simulink library "powerlib_extras"  (Simulink 6.0)
settings: Solver=ode45  SolverMode=SingleTasking  StartTime=0.0  StopTime=10.0  RelTol=1e-3
values from neighbouring files (symbols this model uses):
  Ts = get(handles.edit1,'string')    [powergui.m]
undefined symbols (not defined in the file or in its folder): Ac, Bc, Cc, Dc, Delay_discrete, dend, DiscIntNeverNeededParam, extra_sc, j, numd, test_alpha
libraries: powerlib2 x112, powerlib_extras x70, simulink_extras x25, simulink x12, powerlib_models x8
(part 6 of 9)

== system powerlib_extras/Measurements/dq0-based Active & Reactive Power ==
  note: 2) Q = 3/2(Vq*Id - Vd*Iq)
  note: 1) P = 3/2(Vd*Id + Vq*Iq + 2*V0*I0)
  note: This block computes the 3-phase instantaneous active and reactive power using the following equations:
  note: Note: Equation 2 is valid only for a balanced and harmonic-free system.
  note: dq0-based active and reactive power computation
  note: Gilbert Sybille, Pierre Giroux
      | Power System Simulation Laboratory
      | IREQ, Hydro-Quebc
  Vdq0 : Inport  Port=1  PortDimensions=3  LatchInput=off
  Idq0 : Inport  Port=2  PortDimensions=3  LatchInput=off
  Demux1 : Demux  Outputs=2
  Demux2 : Demux  Outputs=2
  Mux : Mux  Inputs=2
  Product{1..5} (5 alike) : Product  SaturateOnIntegerOverflow=on  InputSameDT=on
  Selector : Selector  Elements=[1 2]  InputPortWidth=3
  Selector1 : Selector  Elements=[1 2]  InputPortWidth=3
  Selector2 : Selector  Elements=3  InputPortWidth=3
  Selector3 : Selector  Elements=3  InputPortWidth=3
  Sum : Sum  Inputs=+++  SaturateOnIntegerOverflow=on  InputSameDT=on
  Sum1 : Sum  Inputs=+-  SaturateOnIntegerOverflow=on  InputSameDT=on
  pu->V1 : Gain  Gain=2  SaturateOnIntegerOverflow=on
  pu->V4 : Gain  Gain=3/2  SaturateOnIntegerOverflow=on
  PQ : Outport
  wires:
  Vdq0/1 -> Selector2/1, Selector/1
  Idq0/1 -> Selector3/1, Selector1/1
  Demux2/2 -> Product3/2, Product5/2
  Demux1/1 -> Product2/1, Product5/1
  Demux2/1 -> Product2/2, Product4/2
  Demux1/2 -> Product3/1, Product4/1
  Sum1/1 -> Mux/2
  Sum/1 -> Mux/1
  Product5/1 -> Sum1/2
  Product4/1 -> Sum1/1
  Product3/1 -> Sum/2
  Product2/1 -> Sum/1
  Selector/1 -> Demux1/1
  Selector1/1 -> Demux2/1
  Selector2/1 -> Product1/1
  Selector3/1 -> Product1/2
  Product1/1 -> pu->V1/1
  pu->V1/1 -> Sum/3
  Mux/1 -> pu->V4/1
  pu->V4/1 -> PQ/1

== system powerlib_extras/Measurements/dq0_to_abc Transformation ==
  note: Va= Vd*sinwt + Vq*cos(wt) + Vo
  note: Vb= Vd*sin(wt-2pi/3) + Vq*cos(wt-2pi/3) + Vo
  note: Vc= Vd*sin(wt+2pi/3) + Vq*cos(wt+2pi/3) + Vo
  dq0 : Inport  Port=1  PortDimensions=3  LatchInput=off
  sin_cos : Inport  Port=2  PortDimensions=2  LatchInput=off
  Demux : Demux  Outputs=2
  Fcn2 : Fcn  Expr="u[1]*u[4] +  u[2]*u[5] + u[3]"
  Fcn4 : Fcn  Expr="u[1]*u[6] +  u[2]*u[7]+ u[3]"
  Fcn5 : Fcn  Expr="u[1]*u[8]+  u[2]*u[9]+ u[3]"
  K1 : Constant  Value=0.5
  K2 : Constant  Value=sqrt(3)/2
  Mux : Mux  Inputs=2
  Mux1 : Mux  Inputs=3
  Mux2 : Mux  Inputs=6
  Product{,1..3} (4 alike) : Product  SaturateOnIntegerOverflow=on  InputSameDT=on
  Sum : Sum  Inputs=--  SaturateOnIntegerOverflow=on  InputSameDT=on
  Sum1 : Sum  Inputs=-+  SaturateOnIntegerOverflow=on  InputSameDT=on
  Sum2 : Sum  Inputs=--  SaturateOnIntegerOverflow=on  InputSameDT=on
  Sum3 : Sum  Inputs=--  SaturateOnIntegerOverflow=on  InputSameDT=on
  abc : Outport  InitialOutput=0
  wires:
  Fcn5/1 -> Mux1/3  "Vc"
  Fcn2/1 -> Mux1/1  "Va"
  Mux1/1 -> abc/1
  Mux/1 -> Fcn4/1, Fcn2/1, Fcn5/1
  Sum1/1 -> Sum3/1, Mux2/4  "cos(wt-2pi/3)"
  Sum/1 -> Sum2/1, Mux2/3  "sin(wt-2pi/3)"
  K2/1 -> Product2/2, Product1/2
  K1/1 -> Product3/2, Product/2
  Sum2/1 -> Mux2/5  "sin(wt+2pi/3)"
  Sum3/1 -> Mux2/6  "cos(wt+2pi/3)"
  Product2/1 -> Sum1/2
  Product3/1 -> Sum1/1
  Product1/1 -> Sum/2
  Product/1 -> Sum/1
  Demux/1 -> Mux2/1, Sum2/2, Product2/1, Product/1  "sin(wt)"
  Demux/2 -> Mux2/2, Product1/1, Product3/1, Sum3/2  "cos(wt)"
  sin_cos/1 -> Demux/1
  Mux2/1 -> Mux/2
  dq0/1 -> Mux/1  "Vabc"
  Fcn4/1 -> Mux1/2  "Vb"

== system powerlib_extras/Phasor Library/3-Phase Active & Reactive Power (Phasor Type) ==
  Vabc : Inport  Port=1  PortDimensions=3  LatchInput=off
  Iabc : Inport  Port=2  PortDimensions=3  LatchInput=off
  Complex to Real-Imag : ComplexToRealImag
  K : Gain  Gain=1/2  SaturateOnIntegerOverflow=on
  Math Function : Math  Operator=conj  SaturateOnIntegerOverflow=on
  Mux : Mux  Inputs=2
  Product2 : Product  SaturateOnIntegerOverflow=on  InputSameDT=on
  Sum3 : Sum  Inputs=1  SaturateOnIntegerOverflow=on  InputSameDT=on
  PQ : Outport
  wires:
  Iabc/1 -> Math Function/1
  Vabc/1 -> Product2/1
  Math Function/1 -> Product2/2
  Product2/1 -> Sum3/1
  Sum3/1 -> K/1
  K/1 -> Complex to Real-Imag/1
  Complex to Real-Imag/1 -> Mux/1
  Complex to Real-Imag/2 -> Mux/2
  Mux/1 -> PQ/1

== system powerlib_extras/Phasor Library/Active & Reactive Power (Phasor Type) ==
  V : Inport  Port=1  LatchInput=off
  I : Inport  Port=2  LatchInput=off
  Complex to Real-Imag : ComplexToRealImag
  K : Gain  Gain=1/2  SaturateOnIntegerOverflow=on
  Math Function : Math  Operator=conj  SaturateOnIntegerOverflow=on
  Mux : Mux  Inputs=2
  Product2 : Product  SaturateOnIntegerOverflow=on  InputSameDT=on
  PQ : Outport
  wires:
  I/1 -> Math Function/1
  K/1 -> Complex to Real-Imag/1
  Product2/1 -> K/1
  Math Function/1 -> Product2/2
  V/1 -> Product2/1
  Complex to Real-Imag/1 -> Mux/1
  Complex to Real-Imag/2 -> Mux/2
  Mux/1 -> PQ/1

== system powerlib_extras/Phasor Library/Mean Value (Phasor Type) ==
  note: Mean value (phasor type)
  In : Inport  Port=1  LatchInput=off
  Complex to Real-Imag : ComplexToRealImag
  Demux : Demux  Outputs=2
  Gain : Gain  Gain=1/Period  SaturateOnIntegerOverflow=on
  Mux : Mux  Inputs=2
  Real-Imag to Complex : RealImagToComplex
  Sum : Sum  Inputs=+-  SaturateOnIntegerOverflow=on  InputSameDT=on
  Transport Delay : TransportDelay  DelayTime=Period
  integrator : Integrator
  Mean : Outport
  wires:
  integrator/1 -> Transport Delay/1, Sum/1
  In/1 -> Complex to Real-Imag/1
  Complex to Real-Imag/1 -> Mux/1
  Complex to Real-Imag/2 -> Mux/2
  Gain/1 -> Demux/1
  Demux/1 -> Real-Imag to Complex/1
  Demux/2 -> Real-Imag to Complex/2
  Real-Imag to Complex/1 -> Mean/1
  Mux/1 -> integrator/1
  Transport Delay/1 -> Sum/2
  Sum/1 -> Gain/1

== system powerlib_extras/Phasor Library/Sequence Analyzer (Phasor Type) ==
  note: Negative sequence :V2 = 1/3 * (Va + a^2*Vb + a *Vc )
  note: Positive sequence :V1 = 1/3 * (Va + a*Vb + a^2 *Vc )
  note: where a =exp(j *2pi/3) = 1 < + 120 deg.
  note: Zero sequence :V0 = 1/3 * (Va + Vb + Vc )
  abc : Inport  Port=1  PortDimensions=3  LatchInput=off
  Complex to Magnitude-Angle : ComplexToMagnitudeAngle
  Constant : Constant  Value=PosOn
  Constant1 : Constant  Value=NegOn
  Constant2 : Constant  Value=ZeroOn
  Mux2 : Mux  Inputs=3
  Neg. Seq. Computation : Subsystem  TreatAsAtomicUnit=on
  Pos. Seq. Computation : Subsystem  TreatAsAtomicUnit=on
  Selector : Selector  Elements=SelectElement  InputPortWidth=3
  Selector1 : Selector  Elements=SelectElement  InputPortWidth=3
  Zero Seq. Computation : Subsystem  TreatAsAtomicUnit=on
  rad->deg1 : Gain  Gain=180/pi  SaturateOnIntegerOverflow=on
  Mag : Outport
  Pha : Outport  Port=2
  wires:
  Constant1/1 -> Neg. Seq. Computation/Enable
  Selector1/1 -> rad->deg1/1
  Constant2/1 -> Zero Seq. Computation/Enable
  Constant/1 -> Pos. Seq. Computation/Enable
  Mux2/1 -> Complex to Magnitude-Angle/1
  Zero Seq. Computation/1(Out) -> Mux2/3
  Neg. Seq. Computation/1(Out) -> Mux2/2
  Pos. Seq. Computation/1(Out) -> Mux2/1
  abc/1 -> Zero Seq. Computation/1(In), Neg. Seq. Computation/1(In), Pos. Seq. Computation/1(In)  "Vabc"
  rad->deg1/1 -> Pha/1
  Selector/1 -> Mag/1
  Complex to Magnitude-Angle/1 -> Selector/1
  Complex to Magnitude-Angle/2 -> Selector1/1

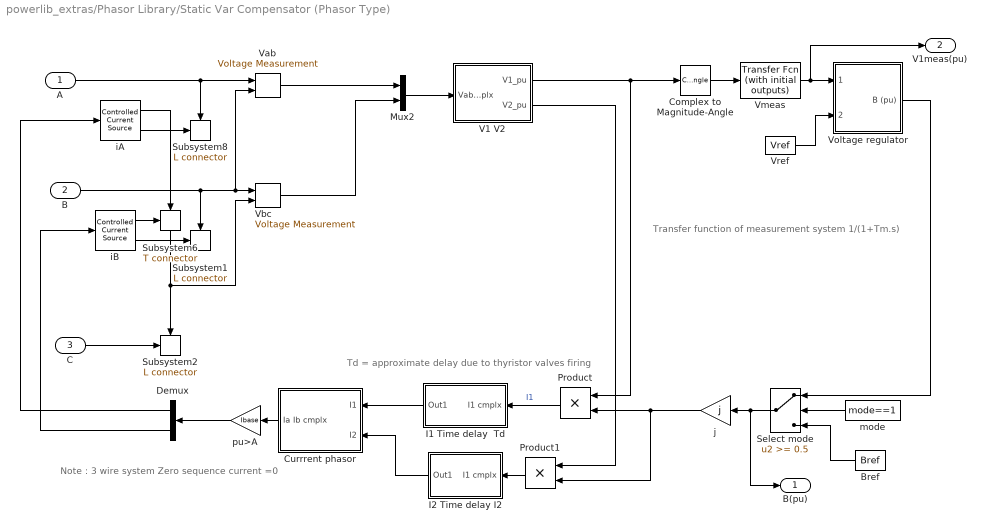
== system powerlib_extras/Phasor Library/Static Var Compensator (Phasor Type) ==
  note: Transfer function of measurement system
      | 1/(1+Tm.s)
  note: Td = approximate delay
      | due to thyristor valves firing
  note: Note : 3 wire system
      | Zero sequence current =0
  A : Inport  Port=1  LatchInput=off
  B : Inport  Port=2  LatchInput=off
  C : Inport  Port=3  LatchInput=off
  Bref : Constant  Orientation=left  Value=Bref
  Complex to Magnitude-Angle : ComplexToMagnitudeAngle  Output=Magnitude
  Currrent phasor : Subsystem  Orientation=left
  Demux : Demux  Orientation=left  Outputs=2
  I1 Time delay  Td : Subsystem  Orientation=left
  I2 Time delay I2 : Subsystem  Orientation=left
  Mux2 : Mux  Inputs=2
  Product : Product  Orientation=left  SaturateOnIntegerOverflow=on  InputSameDT=on
  Product1 : Product  Orientation=left  SaturateOnIntegerOverflow=on  InputSameDT=on
  Select mode : Switch  Orientation=left  Threshold=0.5  InputSameDT=on
  Subsystem1 : powerlib2/Connectors/L connector  Tag=PoWeRsYsTeMbLoCk
  Subsystem2 : powerlib2/Connectors/L connector  Tag=PoWeRsYsTeMbLoCk
  Subsystem6 : powerlib2/Connectors/T connector  Tag=PoWeRsYsTeMbLoCk  Orientation=down  PSBOutputType=1
  Subsystem8 : powerlib2/Connectors/L connector  Tag=PoWeRsYsTeMbLoCk
  V1 V2 : Subsystem
  Vab : powerlib2/Measurements/Voltage Measurement  Tag=PoWeRsYsTeMmEaSuReMeNt  PhasorSimulation=on  OutputType=Complex  PSBOutputType=0  PSBequivalent=0
  Vbc : powerlib2/Measurements/Voltage Measurement  Tag=PoWeRsYsTeMmEaSuReMeNt  PhasorSimulation=on  OutputType=Complex  PSBOutputType=0  PSBequivalent=0
  Vmeas : simulink_extras/Additional Linear/Transfer Fcn (with initial outputs)  N=[1]  D="[Tm  1]"  Y0=Vref  U0=Vref
  Voltage regulator : Subsystem
  Vref : Constant  Value=Vref
  iA : powerlib2/Electrical Sources/Controlled Current Source  Tag=PoWeRsYsTeMbLoCk  Description=source block  initsrc=on  srctyp=AC  ia=0  iph=0  freq=60  mesure=None  PSBOutputType=11
  iB : powerlib2/Electrical Sources/Controlled Current Source  Tag=PoWeRsYsTeMbLoCk  Description=source block  initsrc=on  srctyp=AC  ia=0  iph=0  freq=60  mesure=None  PSBOutputType=11
  j : Gain  Orientation=left  Gain=j  SaturateOnIntegerOverflow=on
  mode : Constant  Orientation=left  Value=mode==1
  pu>A : Gain  Orientation=left  Gain=Ibase  SaturateOnIntegerOverflow=on
  B(pu) : Outport
  V1meas(pu) : Outport  Port=2
  wires:
  mode/1 -> Select mode/2
  Voltage regulator/1(B (pu)) -> Select mode/1
  Bref/1 -> Select mode/3
  Select mode/1 -> B(pu)/1, j/1
  iA/2 -> Subsystem8/1
  A/1 -> Subsystem8/Enable, Vab/1
  iB/2 -> Subsystem1/1
  B/1 -> Subsystem1/Enable, Vab/2, Vbc/1
  iA/1 -> Subsystem6/1
  iB/1 -> Subsystem6/Enable
  Subsystem6/1 -> Subsystem2/Enable, Vbc/2
  C/1 -> Subsystem2/1
  Mux2/1 -> V1 V2/1(Vab Vbc cmplx)
  V1 V2/1(V1_pu) -> Complex to Magnitude-Angle/1, Product/1
  Vref/1 -> Voltage regulator/2(Vref (pu))
  Vmeas/1 -> Voltage regulator/1(V1meas (pu)), V1meas(pu)/1
  Currrent phasor/1(Ia Ib cmplx) -> pu>A/1
  I2 Time delay I2/1(Out1) -> Currrent phasor/2(I2)
  Complex to Magnitude-Angle/1 -> Vmeas/1
  Demux/1 -> iA/1
  Demux/2 -> iB/1
  Vab/1 -> Mux2/1
  Vbc/1 -> Mux2/2
  I1 Time delay  Td/1(Out1) -> Currrent phasor/1(I1)
  pu>A/1 -> Demux/1
  Product/1 -> I1 Time delay  Td/1(I1 cmplx)  "I1"
  j/1 -> Product/2, Product1/2
  V1 V2/2(V2_pu) -> Product1/1
  Product1/1 -> I2 Time delay I2/1(I1 cmplx)

== system powerlib_extras/Three-Phase Library/6 - pulse  diode  bridge ==
  A : Inport  Port=1  LatchInput=off
  B : Inport  Port=2  LatchInput=off
  C : Inport  Port=3  LatchInput=off
  Bus Bar 5 : powerlib2/Connectors/Bus Bar (thin vert)  Tag=PoWeRsYsTeMbLoCk  input=0  output=2  PSBOutputType=111111111111111111111111111111111111111111111111111111111111111111111111111111111111
  D{1..6} (6 alike) : powerlib2/Power Electronics/Diode  Tag=PoWeRsYsTeMbLoCk  Orientation=up  Ron=Ron  Lon=Lon  Vf=Vf  IC=0  Rs=Rs  Cs=Cs  PSBOutputType=10
  Subsystem11 : powerlib2/Connectors/T connector  Tag=PoWeRsYsTeMbLoCk  PSBOutputType=1
  Subsystem12 : powerlib2/Connectors/T connector  Tag=PoWeRsYsTeMbLoCk  PSBOutputType=1
  Subsystem6 : powerlib2/Connectors/T connector  Tag=PoWeRsYsTeMbLoCk  Orientation=up  PSBOutputType=1
  Subsystem7 : powerlib2/Connectors/T connector  Tag=PoWeRsYsTeMbLoCk  Orientation=up  PSBOutputType=1
  Subsystem8 : powerlib2/Connectors/T connector  Tag=PoWeRsYsTeMbLoCk  Orientation=up  PSBOutputType=1
  Terminator{,1..5} (6 alike) : Terminator
      settings: Orientation=up
  "K " : Outport  InitialOutput=0
  "A " : Outport  Port=2  InitialOutput=0
  wires:
  Bus Bar 5/2 -> "A "/1, D2/1, D6/1
  Bus Bar 5/1 -> D4/1
  D4/2 -> Terminator3/1
  D6/2 -> Terminator4/1
  D2/2 -> Terminator5/1
  D5/2 -> Terminator2/1
  D3/2 -> Terminator1/1
  D1/2 -> Terminator/1
  Subsystem12/1 -> "K "/1
  D5/1 -> Subsystem12/Enable
  Subsystem11/1 -> Subsystem12/1
  D3/1 -> Subsystem11/Enable
  D1/1 -> Subsystem11/1
  D6/1 -> Subsystem7/1
  D4/1 -> Subsystem6/1
  C/1 -> Subsystem8/Enable
  Subsystem6/1 -> D1/1
  Subsystem7/1 -> D3/1
  D2/1 -> Subsystem8/1
  Subsystem8/1 -> D5/1
  A/1 -> Subsystem6/Enable
  B/1 -> Subsystem7/Enable

== system powerlib_extras/Three-Phase Library/6 - pulse  thyristor bridge ==
  A : Inport  Port=1  LatchInput=off
  B : Inport  Port=2  LatchInput=off
  C : Inport  Port=3  LatchInput=off
  pulses : Inport  Port=4  LatchInput=off
  Bus Bar 5 : powerlib2/Connectors/Bus Bar (thin vert)  Tag=PoWeRsYsTeMbLoCk  input=0  output=2  PSBOutputType=111111111111111111111111111111111111111111111111111111111111111111111111111111111111
  Demux1 : Demux  Outputs=3
  Demux2 : Demux  Outputs=3
  Selector : Selector  Elements=[ 4 6 2]  InputPortWidth=6
  Selector1 : Selector  Elements=[ 1 3 5]  InputPortWidth=6
  Subsystem14 : powerlib2/Connectors/T connector  Tag=PoWeRsYsTeMbLoCk  PSBOutputType=1
  Subsystem15 : powerlib2/Connectors/T connector  Tag=PoWeRsYsTeMbLoCk  PSBOutputType=1
  Subsystem6 : powerlib2/Connectors/T connector  Tag=PoWeRsYsTeMbLoCk  Orientation=up  PSBOutputType=1
  Subsystem7 : powerlib2/Connectors/T connector  Tag=PoWeRsYsTeMbLoCk  Orientation=up  PSBOutputType=1
  Subsystem8 : powerlib2/Connectors/T connector  Tag=PoWeRsYsTeMbLoCk  Orientation=up  PSBOutputType=1
  Terminator{,1..5} (6 alike) : Terminator
      settings: Orientation=up
  th{1..6} (6 alike) : powerlib2/Power Electronics/Thyristor  Tag=PoWeRsYsTeMbLoCk  Orientation=up  Ron=Ron  Lon=Lon  Vf=0  IC=0  Rs=Rs  Cs=Cs  PSBOutputType=10
  "K " : Outport  InitialOutput=0
  "A " : Outport  Port=2  InitialOutput=0
  wires:
  Bus Bar 5/2 -> "A "/1, th2/1, th6/1
  Bus Bar 5/1 -> th4/1
  Subsystem6/1 -> th1/1
  th4/1 -> Subsystem6/1
  A/1 -> Subsystem6/Enable
  th4/2 -> Terminator3/1
  th6/2 -> Terminator4/1
  th2/2 -> Terminator5/1
  th5/2 -> Terminator2/1
  th3/2 -> Terminator1/1
  th1/2 -> Terminator/1
  Subsystem15/1 -> "K "/1
  th5/1 -> Subsystem15/Enable
  Subsystem14/1 -> Subsystem15/1
  th3/1 -> Subsystem14/Enable
  th1/1 -> Subsystem14/1
  th6/1 -> Subsystem7/1
  pulses/1 -> Selector/1, Selector1/1
  B/1 -> Subsystem7/Enable
  th2/1 -> Subsystem8/1
  Subsystem7/1 -> th3/1
  Demux1/3 -> th5/2
  Demux1/2 -> th3/2
  Demux1/1 -> th1/2
  Selector1/1 -> Demux1/1
  Demux2/3 -> th2/2
  Demux2/2 -> th6/2
  Demux2/1 -> th4/2
  Selector/1 -> Demux2/1
  C/1 -> Subsystem8/Enable
  Subsystem8/1 -> th5/1

== system powerlib_extras/Three-Phase Library/DYg linear transformer ==
  A1 : Inport  Port=1  LatchInput=off
  B1 : Inport  Port=2  LatchInput=off
  C1 : Inport  Port=3  LatchInput=off
  Ground : powerlib2/Connectors/Ground (input)  Tag=PoWeRsYsTeMbLoCk  Orientation=down
  Ground1 : powerlib2/Connectors/Ground (input)  Tag=PoWeRsYsTeMbLoCk  Orientation=down
  Ground2 : powerlib2/Connectors/Ground (input)  Tag=PoWeRsYsTeMbLoCk  Orientation=down
  T1 : powerlib2/Elements/Linear Transformer  Tag=PoWeRsYsTeMbLoCk  a=[pnom fnom]  b=[ u1 r1 x1]  c=[u2 r2 x2]  w3check=off  d=[u2 r2 x2]  e=rxm  mesure=None  PSBOutputType=1111
  T2 : powerlib2/Elements/Linear Transformer  Tag=PoWeRsYsTeMbLoCk  a=[pnom fnom]  b=[ u1 r1 x1]  c=[u2 r2 x2]  w3check=off  d=[u2 r2 x2]  e=rxm  mesure=None  PSBOutputType=1111
  T3 : powerlib2/Elements/Linear Transformer  Tag=PoWeRsYsTeMbLoCk  a=[pnom fnom]  b=[ u1 r1 x1]  c=[u2 r2 x2]  w3check=off  d=[u2 r2 x2]  e=rxm  mesure=None  PSBOutputType=1111
  A2 : Outport  InitialOutput=0
  B2 : Outport  Port=2  InitialOutput=0
  C2 : Outport  Port=3  InitialOutput=0
  wires:
  T1/2 -> Ground/1
  T3/2 -> Ground2/1
  T2/2 -> Ground1/1
  T3/1 -> C2/1
  T2/1 -> B2/1
  T1/1 -> A2/1
  B1/1 -> T1/2, T2/1
  A1/1 -> T3/2, T1/1
  C1/1 -> T2/2, T3/1

== system powerlib_extras/Three-Phase Library/Inductive source with neutral ==
  N : Inport  Port=1  LatchInput=off
  Branch A : powerlib2/Elements/Series RLC Branch  Tag=PoWeRsYsTeMbLoCk  a=R  b=L  c=inf  mesure=None  PSBOutputType=1
  Branch B : powerlib2/Elements/Series RLC Branch  Tag=PoWeRsYsTeMbLoCk  a=R  b=L  c=inf  mesure=None  PSBOutputType=1
  Branch C : powerlib2/Elements/Series RLC Branch  Tag=PoWeRsYsTeMbLoCk  a=R  b=L  c=inf  mesure=None  PSBOutputType=1
  Va : powerlib2/Electrical Sources/AC Voltage Source  Tag=PoWeRsYsTeMbLoCk  A=V  P=Phi  F=F  stime=0  mesure=None  PSBOutputType=1
  Vb : powerlib2/Electrical Sources/AC Voltage Source  Tag=PoWeRsYsTeMbLoCk  A=V  P=Phi-120  F=F  stime=0  mesure=None  PSBOutputType=1
  Vc : powerlib2/Electrical Sources/AC Voltage Source  Tag=PoWeRsYsTeMbLoCk  A=V  P=Phi+120  F=F  stime=0  mesure=None  PSBOutputType=1
  A : Outport
  B : Outport  Port=2
  C : Outport  Port=3
  wires:
  Branch A/1 -> A/1
  Branch B/1 -> B/1
  Branch C/1 -> C/1
  N/1 -> Vb/1, Va/1, Vc/1
  Va/1 -> Branch A/1
  Vb/1 -> Branch B/1
  Vc/1 -> Branch C/1

== system powerlib_extras/Three-Phase Library/YgD  linear transformer  ==
  A1 : Inport  Port=1  LatchInput=off
  B1 : Inport  Port=2  LatchInput=off
  C1 : Inport  Port=3  LatchInput=off
  Subsystem10 : powerlib2/Connectors/T connector  Tag=PoWeRsYsTeMbLoCk  PSBOutputType=1
  Subsystem11 : powerlib2/Connectors/T connector  Tag=PoWeRsYsTeMbLoCk  PSBOutputType=1
  Subsystem9 : powerlib2/Connectors/T connector  Tag=PoWeRsYsTeMbLoCk  PSBOutputType=1
  T1 : powerlib2/Elements/Linear Transformer  Tag=PoWeRsYsTeMbLoCk  a=[pnom fnom]  b=[ u1 r1 x1]  c=[u2 r2 x2]  w3check=off  d=[u2 r2 x2]  e=rxm  mesure=None  PSBOutputType=1111
  T2 : powerlib2/Elements/Linear Transformer  Tag=PoWeRsYsTeMbLoCk  a=[pnom fnom]  b=[ u1 r1 x1]  c=[u2 r2 x2]  w3check=off  d=[u2 r2 x2]  e=rxm  mesure=None  PSBOutputType=1111
  T3 : powerlib2/Elements/Linear Transformer  Tag=PoWeRsYsTeMbLoCk  a=[pnom fnom]  b=[ u1 r1 x1]  c=[u2 r2 x2]  w3check=off  d=[u2 r2 x2]  e=rxm  mesure=None  PSBOutputType=1111
  output Ground1 : powerlib2/Connectors/Ground (output)  Tag=PoWeRsYsTeMbLoCk  Orientation=up  PSBOutputType=1
  output Ground2 : powerlib2/Connectors/Ground (output)  Tag=PoWeRsYsTeMbLoCk  Orientation=up  PSBOutputType=1
  output Ground3 : powerlib2/Connectors/Ground (output)  Tag=PoWeRsYsTeMbLoCk  Orientation=up  PSBOutputType=1
  A2 : Outport  InitialOutput=0
  B2 : Outport  Port=2  InitialOutput=0
  C2 : Outport  Port=3  InitialOutput=0
  wires:
  B1/1 -> T2/1
  C1/1 -> T3/1
  T1/1 -> Subsystem11/1
  T2/1 -> Subsystem10/1
  T1/2 -> Subsystem10/Enable
  T3/1 -> Subsystem9/1
  T2/2 -> Subsystem9/Enable
  T3/2 -> Subsystem11/Enable
  Subsystem11/1 -> A2/1
  Subsystem10/1 -> B2/1
  Subsystem9/1 -> C2/1
  A1/1 -> T1/1
  output Ground1/1 -> T1/2
  output Ground2/1 -> T2/2
  output Ground3/1 -> T3/2

== system powerlib_extras/Three-Phase Library/YgY linear transformer  ==
  A1 : Inport  Port=1  LatchInput=off
  B1 : Inport  Port=2  LatchInput=off
  C1 : Inport  Port=3  LatchInput=off
  Subsystem6 : powerlib2/Connectors/T connector  Tag=PoWeRsYsTeMbLoCk  Orientation=up  PSBOutputType=1
  Subsystem8 : powerlib2/Connectors/L connector  Tag=PoWeRsYsTeMbLoCk  Orientation=up
  T1 : powerlib2/Elements/Linear Transformer  Tag=PoWeRsYsTeMbLoCk  a=[pnom fnom]  b=[ u1 r1 x1]  c=[u2 r2 x2]  w3check=off  d=[u2 r2 x2]  e=rxm  mesure=None  PSBOutputType=1111
  T2 : powerlib2/Elements/Linear Transformer  Tag=PoWeRsYsTeMbLoCk  a=[pnom fnom]  b=[ u1 r1 x1]  c=[u2 r2 x2]  w3check=off  d=[u2 r2 x2]  e=rxm  mesure=None  PSBOutputType=1111
  T3 : powerlib2/Elements/Linear Transformer  Tag=PoWeRsYsTeMbLoCk  a=[pnom fnom]  b=[ u1 r1 x1]  c=[u2 r2 x2]  w3check=off  d=[u2 r2 x2]  e=rxm  mesure=None  PSBOutputType=1111
  output Ground1 : powerlib2/Connectors/Ground (output)  Tag=PoWeRsYsTeMbLoCk  Orientation=up  PSBOutputType=1
  output Ground2 : powerlib2/Connectors/Ground (output)  Tag=PoWeRsYsTeMbLoCk  Orientation=up  PSBOutputType=1
  output Ground3 : powerlib2/Connectors/Ground (output)  Tag=PoWeRsYsTeMbLoCk  Orientation=up  PSBOutputType=1
  A2 : Outport  InitialOutput=0
  B2 : Outport  Port=2  InitialOutput=0
  C2 : Outport  Port=3  InitialOutput=0
  wires:
  T3/1 -> C2/1
  B1/1 -> T2/1
  C1/1 -> T3/1
  T1/1 -> A2/1
  T2/1 -> B2/1
  A1/1 -> T1/1
  output Ground1/1 -> T1/2
  output Ground2/1 -> T2/2
  output Ground3/1 -> T3/2
  T2/2 -> Subsystem6/Enable
  T3/2 -> Subsystem6/1
  T1/2 -> Subsystem8/Enable
  Subsystem6/1 -> Subsystem8/1

== system powerlib_extras/Three-Phase Library/YgYD linear transformer ==
  A1 : Inport  Port=1  LatchInput=off
  B1 : Inport  Port=2  LatchInput=off
  C1 : Inport  Port=3  LatchInput=off
  Subsystem10 : powerlib2/Connectors/L connector  Tag=PoWeRsYsTeMbLoCk
  Subsystem11 : powerlib2/Connectors/T connector  Tag=PoWeRsYsTeMbLoCk  PSBOutputType=1
  Subsystem12 : powerlib2/Connectors/T connector  Tag=PoWeRsYsTeMbLoCk  Orientation=down  PSBOutputType=1
  Subsystem7 : powerlib2/Connectors/T connector  Tag=PoWeRsYsTeMbLoCk  PSBOutputType=1
  Subsystem8 : powerlib2/Connectors/T connector  Tag=PoWeRsYsTeMbLoCk  PSBOutputType=1
  T1 : powerlib2/Elements/Linear Transformer  Tag=PoWeRsYsTeMbLoCk  a=[pnom fnom]  b=[ u1 r1 x1]  c=[u2 r2 x2]  w3check=on  d=[u3 r3 x3]  e=rxm  mesure=None  PSBOutputType=1111
  T2 : powerlib2/Elements/Linear Transformer  Tag=PoWeRsYsTeMbLoCk  a=[pnom fnom]  b=[ u1 r1 x1]  c=[u2 r2 x2]  w3check=on  d=[u3 r3 x3]  e=rxm  mesure=None  PSBOutputType=1111
  T3 : powerlib2/Elements/Linear Transformer  Tag=PoWeRsYsTeMbLoCk  a=[pnom fnom]  b=[ u1 r1 x1]  c=[u2 r2 x2]  w3check=on  d=[u3 r3 x3]  e=rxm  mesure=None  PSBOutputType=1111
  output Ground4 : powerlib2/Connectors/Ground (output)  Tag=PoWeRsYsTeMbLoCk  Orientation=up  PSBOutputType=1
  output Ground5 : powerlib2/Connectors/Ground (output)  Tag=PoWeRsYsTeMbLoCk  Orientation=up  PSBOutputType=1
  output Ground6 : powerlib2/Connectors/Ground (output)  Tag=PoWeRsYsTeMbLoCk  Orientation=up  PSBOutputType=1
  A2 : Outport  InitialOutput=0
  B2 : Outport  Port=2  InitialOutput=0
  C2 : Outport  Port=3  InitialOutput=0
  A3 : Outport  Port=4  InitialOutput=0
  B3 : Outport  Port=5  InitialOutput=0
  C3 : Outport  Port=6  InitialOutput=0
  wires:
  T1/3 -> Subsystem11/1
  Subsystem8/1 -> C3/1
  Subsystem7/1 -> B3/1
  Subsystem11/1 -> A3/1
  T3/3 -> Subsystem8/1
  T2/4 -> Subsystem8/Enable
  T2/3 -> Subsystem7/1
  T1/4 -> Subsystem7/Enable
  T3/2 -> Subsystem10/1
  C1/1 -> T3/1
  output Ground4/1 -> T3/2
  output Ground5/1 -> T2/2
  T3/1 -> C2/1
  T2/1 -> B2/1
  output Ground6/1 -> T1/2
  B1/1 -> T2/1
  A1/1 -> T1/1
  T1/1 -> A2/1
  T2/2 -> Subsystem12/Enable
  T1/2 -> Subsystem12/1
  Subsystem12/1 -> Subsystem10/Enable
  T3/4 -> Subsystem11/Enable

== system powerlib_extras/Three-Phase Library/YgYgD linear transformer ==
  A1 : Inport  Port=1  LatchInput=off
  B1 : Inport  Port=2  LatchInput=off
  C1 : Inport  Port=3  LatchInput=off
  Ground : powerlib2/Connectors/Ground (input)  Tag=PoWeRsYsTeMbLoCk
  Ground1 : powerlib2/Connectors/Ground (input)  Tag=PoWeRsYsTeMbLoCk
  Ground2 : powerlib2/Connectors/Ground (input)  Tag=PoWeRsYsTeMbLoCk
  Subsystem7 : powerlib2/Connectors/T connector  Tag=PoWeRsYsTeMbLoCk  PSBOutputType=1
  Subsystem8 : powerlib2/Connectors/T connector  Tag=PoWeRsYsTeMbLoCk  PSBOutputType=1
  Subsystem9 : powerlib2/Connectors/T connector  Tag=PoWeRsYsTeMbLoCk  PSBOutputType=1
  T1 : powerlib2/Elements/Linear Transformer  Tag=PoWeRsYsTeMbLoCk  a=[pnom fnom]  b=[ u1 r1 x1]  c=[u2 r2 x2]  w3check=on  d=[u3 r3 x3]  e=rxm  mesure=None  PSBOutputType=1111
  T2 : powerlib2/Elements/Linear Transformer  Tag=PoWeRsYsTeMbLoCk  a=[pnom fnom]  b=[ u1 r1 x1]  c=[u2 r2 x2]  w3check=on  d=[u3 r3 x3]  e=rxm  mesure=None  PSBOutputType=1111
  T3 : powerlib2/Elements/Linear Transformer  Tag=PoWeRsYsTeMbLoCk  a=[pnom fnom]  b=[ u1 r1 x1]  c=[u2 r2 x2]  w3check=on  d=[u3 r3 x3]  e=rxm  mesure=None  PSBOutputType=1111
  output Ground3 : powerlib2/Connectors/Ground (output)  Tag=PoWeRsYsTeMbLoCk  Orientation=up  PSBOutputType=1
  output Ground4 : powerlib2/Connectors/Ground (output)  Tag=PoWeRsYsTeMbLoCk  Orientation=up  PSBOutputType=1
  output Ground5 : powerlib2/Connectors/Ground (output)  Tag=PoWeRsYsTeMbLoCk  Orientation=up  PSBOutputType=1
  A2 : Outport  InitialOutput=0
  B2 : Outport  Port=2  InitialOutput=0
  C2 : Outport  Port=3  InitialOutput=0
  A3 : Outport  Port=4  InitialOutput=0
  B3 : Outport  Port=5  InitialOutput=0
  C3 : Outport  Port=6  InitialOutput=0
  wires:
  T3/4 -> Subsystem9/Enable
  T3/3 -> Subsystem8/1
  T2/4 -> Subsystem8/Enable
  T2/3 -> Subsystem7/1
  T3/2 -> Ground2/1
  T2/2 -> Ground1/1
  T3/1 -> C2/1
  T2/1 -> B2/1
  output Ground5/1 -> T3/2
  C1/1 -> T3/1
  B1/1 -> T2/1
  output Ground4/1 -> T2/2
  Subsystem7/1 -> B3/1
  Subsystem8/1 -> C3/1
  T1/4 -> Subsystem7/Enable
  T1/1 -> A2/1
  A1/1 -> T1/1
  T1/2 -> Ground/1
  output Ground3/1 -> T1/2
  Subsystem9/1 -> A3/1
  T1/3 -> Subsystem9/1

== system powerlib_extras/Three-Phase Library/YgYgD saturable transformer ==
  A1 : Inport  Port=1  LatchInput=off
  B1 : Inport  Port=2  LatchInput=off
  C1 : Inport  Port=3  LatchInput=off
  Ground : powerlib2/Connectors/Ground (input)  Tag=PoWeRsYsTeMbLoCk
  Ground1 : powerlib2/Connectors/Ground (input)  Tag=PoWeRsYsTeMbLoCk
  Ground2 : powerlib2/Connectors/Ground (input)  Tag=PoWeRsYsTeMbLoCk
  Subsystem7 : powerlib2/Connectors/T connector  Tag=PoWeRsYsTeMbLoCk  PSBOutputType=1
  Subsystem8 : powerlib2/Connectors/T connector  Tag=PoWeRsYsTeMbLoCk  PSBOutputType=1
  Subsystem9 : powerlib2/Connectors/T connector  Tag=PoWeRsYsTeMbLoCk  PSBOutputType=1
  T1 : powerlib2/Elements/Saturable Transformer  Tag=PoWeRsYsTeMbLoCk  a=[pnom fnom]  b=[u1 r1 x1]  c=[u2 r2 x2]  w3check=on  d=[u3 r3 x3]  e=sat  f=Rm_phi0_1  H=off  matfile='hysteresis'  Initialslope=+1  mesure=None  PSBOutputType=1111
  T2 : powerlib2/Elements/Saturable Transformer  Tag=PoWeRsYsTeMbLoCk  a=[pnom fnom]  b=[u1 r1 x1]  c=[u2 r2 x2]  w3check=on  d=[u3 r3 x3]  e=sat  f=Rm_phi0_2  H=off  matfile='hysteresis'  Initialslope=+1  mesure=None  PSBOutputType=1111
  T3 : powerlib2/Elements/Saturable Transformer  Tag=PoWeRsYsTeMbLoCk  a=[pnom fnom]  b=[u1 r1 x1]  c=[u2 r2 x2]  w3check=on  d=[u3 r3 x3]  e=sat  f=Rm_phi0_3  H=off  matfile='hysteresis'  Initialslope=+1  mesure=None  PSBOutputType=1111
  output Ground3 : powerlib2/Connectors/Ground (output)  Tag=PoWeRsYsTeMbLoCk  Orientation=up  PSBOutputType=1
  output Ground4 : powerlib2/Connectors/Ground (output)  Tag=PoWeRsYsTeMbLoCk  Orientation=up  PSBOutputType=1
  output Ground5 : powerlib2/Connectors/Ground (output)  Tag=PoWeRsYsTeMbLoCk  Orientation=up  PSBOutputType=1
  A2 : Outport  InitialOutput=0
  B2 : Outport  Port=2  InitialOutput=0
  C2 : Outport  Port=3  InitialOutput=0
  A3 : Outport  Port=4  InitialOutput=0
  B3 : Outport  Port=5  InitialOutput=0
  C3 : Outport  Port=6  InitialOutput=0
  wires:
  T3/1 -> C2/1
  T2/1 -> B2/1
  T3/4 -> Subsystem9/Enable
  T3/3 -> Subsystem8/1
  T2/4 -> Subsystem8/Enable
  T2/3 -> Subsystem7/1
  T1/4 -> Subsystem7/Enable
  T1/3 -> Subsystem9/1
  T1/1 -> A2/1
  T3/2 -> Ground2/1
  T2/2 -> Ground1/1
  output Ground5/1 -> T3/2
  C1/1 -> T3/1
  B1/1 -> T2/1
  output Ground4/1 -> T2/2
  Subsystem7/1 -> B3/1
  Subsystem8/1 -> C3/1
  A1/1 -> T1/1
  T1/2 -> Ground/1
  output Ground3/1 -> T1/2
  Subsystem9/1 -> A3/1

== system powerlib_extras/Control  Blocks/ Synchronized 12-Pulse Generator/12 Flip-Flops ==
  S : Inport  Port=1  LatchInput=off
  R : Inport  Port=2  LatchInput=off
  6 Flip-Flop : Subsystem
  6 Flip-Flop1 : Subsystem
  Demux : Demux  Outputs=2
  Demux1 : Demux  Outputs=2
  Mux : Mux  Inputs=2
  Q : Outport
  wires:
  S/1 -> Demux/1
  Demux/1 -> 6 Flip-Flop/1(S)
  Demux/2 -> 6 Flip-Flop1/1(S)
  R/1 -> Demux1/1
  Demux1/2 -> 6 Flip-Flop1/2(R)
  Demux1/1 -> 6 Flip-Flop/2(R)
  6 Flip-Flop/1(Q) -> Mux/1
  Mux/1 -> Q/1
  6 Flip-Flop1/1(Q) -> Mux/2

== system powerlib_extras/Control  Blocks/1-phase  PLL/Discrete PI Controller ==
  Error : Inport  Port=1  LatchInput=off
  Integrator : Integrator  InitialCondition=Init  LimitOutput=on  UpperSaturationLimit=UpperLimit  LowerSaturationLimit=LowerLimit
  Kp4 : Gain  Gain=Kp  SaturateOnIntegerOverflow=on
  Kp5 : Gain  Gain=Ki  SaturateOnIntegerOverflow=on
  Saturation2 : Saturate  UpperLimit=UpperLimit  LowerLimit=LowerLimit
  Sum6 : Sum  SaturateOnIntegerOverflow=on  InputSameDT=on
  Out : Outport  InitialOutput=0
  wires:
  Error/1 -> Kp4/1, Kp5/1
  Sum6/1 -> Saturation2/1
  Kp5/1 -> Integrator/1
  Kp4/1 -> Sum6/1
  Integrator/1 -> Sum6/2
  Saturation2/1 -> Out/1

== system powerlib_extras/Control  Blocks/1-phase  PLL/Variable Frequency Mean value ==
  Freq : Inport  Port=1  LatchInput=off
  In : Inport  Port=2  LatchInput=off
  Constant : Constant  Value=Vinit
  Integrator : Integrator
  Number of samples per cycle : Fcn  Expr=1/u[1]
  Product : Product  SaturateOnIntegerOverflow=on  InputSameDT=on
  Step : Step  Time=1/Finit  SampleTime=0
  Sum7 : Sum  Inputs=-+  SaturateOnIntegerOverflow=on  InputSameDT=on
  Switch : Switch  Threshold=0.5  InputSameDT=on
  To avoid division by zero : Saturate  Orientation=down  UpperLimit=1e6  LowerLimit=1e-6
  Variable Transport Delay : VariableTransportDelay  MaximumDelay=1/40  MaximumPoints=4096
  Mean : Outport
  wires:
  Number of samples per cycle/1 -> Variable Transport Delay/2  "Delay"
  Step/1 -> Switch/2
  To avoid division by zero/1 -> Number of samples per cycle/1  "Freq"
  Switch/1 -> Mean/1
  Constant/1 -> Switch/3
  Freq/1 -> To avoid division by zero/1, Product/2  "Freq"
  Integrator/1 -> Variable Transport Delay/1, Sum7/2
  Sum7/1 -> Product/1
  Variable Transport Delay/1 -> Sum7/1
  Product/1 -> Switch/1  "Mean value"
  In/1 -> Integrator/1  "In"

== system powerlib_extras/Control  Blocks/3-phase PLL/Discrete PI Controller ==
  Error : Inport  Port=1  LatchInput=off
  Integrator : Integrator  InitialCondition=Init  LimitOutput=on  UpperSaturationLimit=UpperLimit  LowerSaturationLimit=LowerLimit
  Kp4 : Gain  Gain=Kp  SaturateOnIntegerOverflow=on
  Kp5 : Gain  Gain=Ki  SaturateOnIntegerOverflow=on
  Saturation2 : Saturate  UpperLimit=UpperLimit  LowerLimit=LowerLimit
  Sum6 : Sum  SaturateOnIntegerOverflow=on  InputSameDT=on
  Out : Outport  InitialOutput=0
  wires:
  Error/1 -> Kp4/1, Kp5/1
  Sum6/1 -> Saturation2/1
  Kp5/1 -> Integrator/1
  Kp4/1 -> Sum6/1
  Integrator/1 -> Sum6/2
  Saturation2/1 -> Out/1

== system powerlib_extras/Control  Blocks/3-phase PLL/Variable Frequency Mean value ==
  Freq : Inport  Port=1  LatchInput=off
  In : Inport  Port=2  LatchInput=off
  Constant : Constant  Value=Vinit
  Integrator : Integrator
  Number of samples per cycle : Fcn  Expr=1/u[1]
  Product : Product  SaturateOnIntegerOverflow=on  InputSameDT=on
  Step : Step  Time=1/Finit  SampleTime=0
  Sum7 : Sum  Inputs=-+  SaturateOnIntegerOverflow=on  InputSameDT=on
  Switch : Switch  Threshold=0.5  InputSameDT=on
  To avoid division by zero : Saturate  Orientation=down  UpperLimit=1e6  LowerLimit=1e-6
  Variable Transport Delay : VariableTransportDelay  MaximumDelay=1/40  MaximumPoints=4096
  Mean : Outport
  wires:
  Number of samples per cycle/1 -> Variable Transport Delay/2  "Delay"
  Step/1 -> Switch/2
  To avoid division by zero/1 -> Number of samples per cycle/1  "Freq"
  Switch/1 -> Mean/1
  Constant/1 -> Switch/3
  Freq/1 -> To avoid division by zero/1, Product/2  "Freq"
  Integrator/1 -> Variable Transport Delay/1, Sum7/2
  Sum7/1 -> Product/1
  Variable Transport Delay/1 -> Sum7/1
  Product/1 -> Switch/1  "Mean value"
  In/1 -> Integrator/1  "In"

== system powerlib_extras/Control  Blocks/Bistable/RESET Priority ==
  S : Inport  Port=1  LatchInput=off
  R : Inport  Port=2  LatchInput=off
  Enable : EnablePort
  IC=ic : Memory  Orientation=left  X0=ic  InheritSampleTime=on
  Logical Operator : Logic  Operator=OR
  Logical Operator1 : Logic  Operator=NOT  Inputs=1
  Logical Operator2 : Logic
  Logical Operator3 : Logic  Operator=NOT  Inputs=1
  Q : Outport
  !Q : Outport  Port=2
  wires:
  Logical Operator2/1 -> Q/1, Logical Operator3/1, IC=ic/1
  Logical Operator1/1 -> Logical Operator2/2
  R/1 -> Logical Operator1/1
  Logical Operator/1 -> Logical Operator2/1
  IC=ic/1 -> Logical Operator/2
  Logical Operator3/1 -> !Q/1
  S/1 -> Logical Operator/1

== system powerlib_extras/Control  Blocks/Bistable/SET  Priority ==
  S : Inport  Port=1  LatchInput=off
  R : Inport  Port=2  LatchInput=off
  Enable : EnablePort
  IC=ic : Memory  Orientation=left  X0=ic  InheritSampleTime=on
  Logical Operator : Logic  Operator=OR
  Logical Operator1 : Logic  Operator=NOT  Inputs=1
  Logical Operator2 : Logic
  Logical Operator3 : Logic  Operator=NOT  Inputs=1
  Q : Outport
  !Q : Outport  Port=2
  wires:
  Logical Operator2/1 -> Logical Operator/2
  IC=ic/1 -> Logical Operator2/2
  Logical Operator1/1 -> Logical Operator2/1
  R/1 -> Logical Operator1/1
  Logical Operator/1 -> Q/1, Logical Operator3/1, IC=ic/1
  Logical Operator3/1 -> !Q/1
  S/1 -> Logical Operator/1

== system powerlib_extras/Control  Blocks/Edge Detector/NEGATIVE Edge ==
  IN : Inport  Port=1  LatchInput=off
  IN previous : Inport  Port=2  LatchInput=off
  Enable : EnablePort
  Relational Operator1 : RelationalOperator  Operator=>  InputSameDT=on
  OUT : Outport
  wires:
  IN/1 -> Relational Operator1/2
  IN previous/1 -> Relational Operator1/1
  Relational Operator1/1 -> OUT/1

== system powerlib_extras/Control  Blocks/Edge Detector/POSITIVE Edge ==
  IN : Inport  Port=1  LatchInput=off
  IN previous : Inport  Port=2  LatchInput=off
  Enable : EnablePort
  Relational Operator1 : RelationalOperator  Operator=>  InputSameDT=on
  OUT : Outport
  wires:
  IN/1 -> Relational Operator1/1
  IN previous/1 -> Relational Operator1/2
  Relational Operator1/1 -> OUT/1

== system powerlib_extras/Control  Blocks/Monostable/Edge Detector ==
  note: Edge or Slope Detector
  note: Silvano Casoria
      | Power System Simulation Laboratory
      | IREQ, Hydro-Quebc
  In : Inport  Port=1  LatchInput=off
  Constant1 : Constant  Value=model
  Demux : Demux  Outputs=2
  Logical Operator1 : Logic  Operator=OR
  Memory : Memory  X0=ic  InheritSampleTime=on
  Multiport Switch : MultiPortSwitch  Inputs=3  SaturateOnIntegerOverflow=on
  NEGATIVE Edge : Subsystem  AncestorBlock=extra_sc/Edge/POSITIVE Edge  TreatAsAtomicUnit=on
  POSITIVE Edge : Subsystem  AncestorBlock=extra_sc/Delay_discrete/OFF Delay  TreatAsAtomicUnit=on
  either edge : Constant  Value=[1 1]
  neg. edge : Constant  Value=[0 1]
  pos. edge : Constant  Value=[1 0]
  Out : Outport
  wires:
  either edge/1 -> Multiport Switch/4
  Demux/2 -> NEGATIVE Edge/Enable
  Demux/1 -> POSITIVE Edge/Enable
  Multiport Switch/1 -> Demux/1
  Constant1/1 -> Multiport Switch/1
  neg. edge/1 -> Multiport Switch/3
  pos. edge/1 -> Multiport Switch/2
  In/1 -> Memory/1, NEGATIVE Edge/1(IN), POSITIVE Edge/1(IN)
  Memory/1 -> NEGATIVE Edge/2(IN previous), POSITIVE Edge/2(IN previous)
  POSITIVE Edge/1(OUT) -> Logical Operator1/1
  NEGATIVE Edge/1(OUT) -> Logical Operator1/2
  Logical Operator1/1 -> Out/1

== system powerlib_extras/Control  Blocks/On/Off Delay/OFF Delay ==
  note: ic=-inf
  IN : Inport  Port=1  LatchInput=off
  clock : Inport  Port=2  LatchInput=off
  DELAY : Inport  Port=3  LatchInput=off
  Enable : EnablePort
  Edge Detector : powerlib_extras/Control  Blocks/Edge Detector  model=Falling  ic=ic
  Logical Operator : Logic  Operator=NOT  Inputs=1
  Logical Operator1 : Logic  OutDataTypeMode=Boolean
  Logical Operator2 : Logic  Operator=NOT  Inputs=1
  Relational Operator : RelationalOperator  LogicOutDataTypeMode=Boolean  InputSameDT=on
  Sample & Hold : powerlib_extras/Control  Blocks/Sample & Hold  ic=-1e99
  Sum : Sum  SaturateOnIntegerOverflow=on  InputSameDT=on
  OUT : Outport
  wires:
  Edge Detector/1 -> Sample & Hold/2
  clock/1 -> Sample & Hold/1, Relational Operator/1
  Logical Operator/1 -> Logical Operator1/1
  IN/1 -> Edge Detector/1, Logical Operator/1
  Logical Operator2/1 -> OUT/1
  Logical Operator1/1 -> Logical Operator2/1
  Relational Operator/1 -> Logical Operator1/2
  DELAY/1 -> Sum/2
  Sum/1 -> Relational Operator/2
  Sample & Hold/1 -> Sum/1

== system powerlib_extras/Control  Blocks/On/Off Delay/ON Delay ==
  note: ic=-inf
  IN : Inport  Port=1  LatchInput=off
  clock : Inport  Port=2  LatchInput=off
  DELAY : Inport  Port=3  LatchInput=off
  Enable : EnablePort
  Edge Detector : powerlib_extras/Control  Blocks/Edge Detector  model=Rising  ic=ic
  Logical Operator2 : Logic
  Relational Operator : RelationalOperator  LogicOutDataTypeMode=Boolean  InputSameDT=on
  Sample & Hold : powerlib_extras/Control  Blocks/Sample & Hold  ic=-1e99
  Sum : Sum  SaturateOnIntegerOverflow=on  InputSameDT=on
  OUT : Outport
  wires:
  Logical Operator2/1 -> OUT/1
  IN/1 -> Logical Operator2/2, Edge Detector/1
  clock/1 -> Relational Operator/1, Sample & Hold/1
  Sum/1 -> Relational Operator/2
  DELAY/1 -> Sum/2
  Relational Operator/1 -> Logical Operator2/1
  Edge Detector/1 -> Sample & Hold/2
  Sample & Hold/1 -> Sum/1

== system powerlib_extras/Control  Blocks/Synchronized 6-Pulse Generator/6 Flip-Flop ==
  S : Inport  Port=1  LatchInput=off
  R : Inport  Port=2  LatchInput=off
  Demux : Demux  Outputs=6
  Demux1 : Demux  Outputs=6
  Mux : Mux  Inputs=6
  S-R Flip-Flop{1..6} (6 alike) : simulink_extras/Flip Flops/S-R Flip-Flop  initial_condition=0
  Terminator{,1..5} (6 alike) : Terminator
  Q : Outport
  wires:
  S-R Flip-Flop6/2 -> Terminator5/1
  S-R Flip-Flop5/2 -> Terminator4/1
  S-R Flip-Flop4/2 -> Terminator3/1
  S-R Flip-Flop3/2 -> Terminator2/1
  S-R Flip-Flop2/2 -> Terminator1/1
  S-R Flip-Flop1/1 -> Mux/1
  S-R Flip-Flop2/1 -> Mux/2
  S-R Flip-Flop3/1 -> Mux/3
  S-R Flip-Flop4/1 -> Mux/4
  S-R Flip-Flop5/1 -> Mux/5
  Mux/1 -> Q/1
  S-R Flip-Flop6/1 -> Mux/6
  S-R Flip-Flop1/2 -> Terminator/1
  Demux/1 -> S-R Flip-Flop1/1
  Demux/2 -> S-R Flip-Flop2/1
  Demux/3 -> S-R Flip-Flop3/1
  Demux/4 -> S-R Flip-Flop4/1
  S/1 -> Demux/1
  Demux/6 -> S-R Flip-Flop6/1
  Demux/5 -> S-R Flip-Flop5/1
  R/1 -> Demux1/1
  Demux1/1 -> S-R Flip-Flop1/2
  Demux1/2 -> S-R Flip-Flop2/2
  Demux1/3 -> S-R Flip-Flop3/2
  Demux1/4 -> S-R Flip-Flop4/2
  Demux1/5 -> S-R Flip-Flop5/2
  Demux1/6 -> S-R Flip-Flop6/2

== system powerlib_extras/Discrete Measurements/Discrete Variable Frequency Mean value/Correction subsystem ==
  N : Inport  Port=1  LatchInput=off
  F : Inport  Port=2  LatchInput=off
  In : Inport  Port=3  LatchInput=off
  Gain1 : Gain  Gain=0.5  SaturateOnIntegerOverflow=on
  Product2 : Product  Inputs=*/  SaturateOnIntegerOverflow=on  InputSameDT=on
  Product4 : Product  Inputs=**  SaturateOnIntegerOverflow=on  InputSameDT=on
  Product5 : Product  Inputs=**  SaturateOnIntegerOverflow=on  InputSameDT=on
  Sum1 : Sum  Inputs=+-  SaturateOnIntegerOverflow=on  InputSameDT=on
  Sum4 : Sum  SaturateOnIntegerOverflow=on  InputSameDT=on
  Sum5 : Sum  Inputs=+-  SaturateOnIntegerOverflow=on  InputSameDT=on
  Unit Delay : UnitDelay  SampleTime=Ts
  Out : Outport
  wires:
  Product4/1 -> Out/1
  Sum4/1 -> Product4/2
  Gain1/1 -> Sum4/1
  Product5/1 -> Gain1/1
  Sum1/1 -> Product5/2
  In/1 -> Sum4/2, Unit Delay/1, Sum1/1
  Product2/1 -> Product4/1
  Sum5/1 -> Product5/1, Product2/1
  F/1 -> Sum5/2
  N/1 -> Product2/2, Sum5/1
  Unit Delay/1 -> Sum1/2

== system powerlib_extras/Discrete Measurements/Discrete Variable Frequency Mean value/Discrete Variable Transport Delay ==
  In : Inport  Port=1  LatchInput=off
  D : Inport  Port=2  LatchInput=off
  "S-Function " : S-Function  FunctionName=discreteVariableTransportDelay  Parameters=MaxDelay,Ts,InitialValue
  Out : Outport
  wires:
  D/1 -> "S-Function "/2
  In/1 -> "S-Function "/1
  "S-Function "/1 -> Out/1

== system powerlib_extras/Discrete Measurements/Discrete 3-phase Sequence Analyzer/Determine if pha20 are set to zero ==
  Mag120 : Inport  Port=1  LatchInput=off
  Pha120* : Inport  Port=2  LatchInput=off
  Constant4 : Constant  Value=0
  Demux : Demux  Outputs=[1 2]
  K : Gain  Gain=0.002  SaturateOnIntegerOverflow=on
  Mux1 : Mux  Inputs=[1 2]
  Relational Operator : RelationalOperator  Operator=>  InputSameDT=on
  Selector : Selector  Elements=[2 3]  InputPortWidth=3
  Selector2 : Selector  Elements=[1]  InputPortWidth=3
  Switch : Switch  Threshold=0.5  InputSameDT=on
  Pha120 : Outport
  wires:
  K/1 -> Relational Operator/2
  Selector/1 -> Relational Operator/1
  Constant4/1 -> Switch/3
  Selector2/1 -> K/1
  Mag120/1 -> Selector2/1, Selector/1
  Pha120*/1 -> Demux/1
  Mux1/1 -> Pha120/1
  Switch/1 -> Mux1/2
  Demux/2 -> Switch/1
  Demux/1 -> Mux1/1
  Relational Operator/1 -> Switch/2

== system powerlib_extras/Discrete Measurements/Discrete 3-phase Sequence Analyzer/Neg. Seq. Computation ==
  In : Inport  Port=1  LatchInput=off
  Enable : EnablePort
  Gain1 : Gain  Gain=[1 a2 a]  SaturateOnIntegerOverflow=on
  Gain3 : Gain  Gain=1/3  SaturateOnIntegerOverflow=on
  Sum : Sum  Inputs=1  SaturateOnIntegerOverflow=on  InputSameDT=on
  Out : Outport
  wires:
  Gain1/1 -> Sum/1
  Sum/1 -> Gain3/1
  In/1 -> Gain1/1
  Gain3/1 -> Out/1

== system powerlib_extras/Discrete Measurements/Discrete 3-phase Sequence Analyzer/Phasor A ==
  in : Inport  Port=1  LatchInput=off
  sin : Inport  Port=2  LatchInput=off
  cos : Inport  Port=3  LatchInput=off
  "Discrete  Mean value " : powerlib_extras/Discrete Measurements/Discrete  Mean value  Freq=Freq  Vinit=Real_Init  Ts=Ts
  "Discrete  Mean value  " : powerlib_extras/Discrete Measurements/Discrete  Mean value  Freq=Freq  Vinit=Imag_Init  Ts=Ts
  Product2 : Product  SaturateOnIntegerOverflow=on  InputSameDT=on
  Product3 : Product  SaturateOnIntegerOverflow=on  InputSameDT=on
  Real-Imag to Complex : RealImagToComplex
  Out : Outport  InitialOutput=0
  wires:
  sin/1 -> Product2/1
  cos/1 -> Product3/2
  Product2/1 -> "Discrete  Mean value "/1
  Product3/1 -> "Discrete  Mean value  "/1
  in/1 -> Product3/1, Product2/2
  "Discrete  Mean value "/1 -> Real-Imag to Complex/1  "Real"
  "Discrete  Mean value  "/1 -> Real-Imag to Complex/2  "Real"
  Real-Imag to Complex/1 -> Out/1

== system powerlib_extras/Discrete Measurements/Discrete 3-phase Sequence Analyzer/Pos. Seq. Computation ==
  In : Inport  Port=1  LatchInput=off
  Enable : EnablePort
  Gain1 : Gain  Gain=[1 a a2]  SaturateOnIntegerOverflow=on
  Gain3 : Gain  Gain=1/3  SaturateOnIntegerOverflow=on
  Sum : Sum  Inputs=1  SaturateOnIntegerOverflow=on  InputSameDT=on
  Out : Outport
  wires:
  Gain1/1 -> Sum/1
  Sum/1 -> Gain3/1
  In/1 -> Gain1/1
  Gain3/1 -> Out/1

== system powerlib_extras/Discrete Measurements/Discrete 3-phase Sequence Analyzer/Zero Seq. Computation ==
  In : Inport  Port=1  LatchInput=off
  Enable : EnablePort
  Gain3 : Gain  Gain=1/3  SaturateOnIntegerOverflow=on
  Sum : Sum  Inputs=1  SaturateOnIntegerOverflow=on  InputSameDT=on
  Out : Outport
  wires:
  Sum/1 -> Gain3/1
  In/1 -> Sum/1
  Gain3/1 -> Out/1

== system powerlib_extras/Discrete  Control Blocks/Discrete 2nd-Order Variable-Tuned Filter/Predict1 ==
  In : Inport  Port=1  LatchInput=off
  Gain4 : Gain  Gain=2  SaturateOnIntegerOverflow=on
  Sum1 : Sum  Inputs=+-  SaturateOnIntegerOverflow=on  InputSameDT=on
  Unit Delay2 : UnitDelay  X0=VL  SampleTime=Ts
  Out : Outport
  wires:
  Sum1/1 -> Out/1
  In/1 -> Unit Delay2/1, Gain4/1
  Gain4/1 -> Sum1/1
  Unit Delay2/1 -> Sum1/2

== system powerlib_extras/Discrete  Control Blocks/Discrete Bistable/RESET Priority ==
  S : Inport  Port=1  LatchInput=off
  R : Inport  Port=2  LatchInput=off
  Enable : EnablePort
  IC = ic : UnitDelay  Orientation=left  X0=ic  SampleTime=Ts
  Logical Operator : Logic  Operator=OR
  Logical Operator1 : Logic  Operator=NOT  Inputs=1
  Logical Operator2 : Logic
  Logical Operator3 : Logic  Operator=NOT  Inputs=1
  Q : Outport
  !Q : Outport  Port=2
  wires:
  S/1 -> Logical Operator/1
  Logical Operator3/1 -> !Q/1
  IC = ic/1 -> Logical Operator/2
  Logical Operator/1 -> Logical Operator2/1
  R/1 -> Logical Operator1/1
  Logical Operator1/1 -> Logical Operator2/2
  Logical Operator2/1 -> IC = ic/1, Logical Operator3/1, Q/1

== system powerlib_extras/Discrete  Control Blocks/Discrete Bistable/SET  Priority ==
  S : Inport  Port=1  LatchInput=off
  R : Inport  Port=2  LatchInput=off
  Enable : EnablePort
  IC = ic : UnitDelay  Orientation=left  X0=ic  SampleTime=Ts
  Logical Operator : Logic  Operator=OR
  Logical Operator1 : Logic  Operator=NOT  Inputs=1
  Logical Operator2 : Logic
  Logical Operator3 : Logic  Operator=NOT  Inputs=1
  Q : Outport
  !Q : Outport  Port=2
  wires:
  Logical Operator2/1 -> Logical Operator/2
  IC = ic/1 -> Logical Operator2/2
  Logical Operator1/1 -> Logical Operator2/1
  R/1 -> Logical Operator1/1
  Logical Operator/1 -> Q/1, Logical Operator3/1, IC = ic/1
  Logical Operator3/1 -> !Q/1
  S/1 -> Logical Operator/1

== system powerlib_extras/Discrete  Control Blocks/Discrete Edge Detector/NEGATIVE Edge ==
  IN : Inport  Port=1  LatchInput=off
  IN previous : Inport  Port=2  LatchInput=off
  Enable : EnablePort
  Relational Operator1 : RelationalOperator  Operator=>  InputSameDT=on
  OUT : Outport
  wires:
  IN/1 -> Relational Operator1/2
  IN previous/1 -> Relational Operator1/1
  Relational Operator1/1 -> OUT/1

== system powerlib_extras/Discrete  Control Blocks/Discrete Edge Detector/POSITIVE Edge ==
  IN : Inport  Port=1  LatchInput=off
  IN previous : Inport  Port=2  LatchInput=off
  Enable : EnablePort
  Relational Operator1 : RelationalOperator  Operator=>  InputSameDT=on
  OUT : Outport
  wires:
  IN/1 -> Relational Operator1/1
  IN previous/1 -> Relational Operator1/2
  Relational Operator1/1 -> OUT/1

== system powerlib_extras/Discrete  Control Blocks/Discrete Monostable/Edge_Detector ==
  note: Edge or Slope Detector
  note: Silvano Casoria
      | Power System Simulation Laboratory
      | IREQ, Hydro-Quebc
  In : Inport  Port=1  LatchInput=off
  Constant1 : Constant  Value=model
  Demux : Demux  Outputs=2
  Logical Operator1 : Logic  Operator=OR
  Multiport Switch : MultiPortSwitch  Inputs=3  SaturateOnIntegerOverflow=on
  NEGATIVE Edge : Subsystem  AncestorBlock=extra_sc/Edge/POSITIVE Edge  TreatAsAtomicUnit=on
  POSITIVE Edge : Subsystem  AncestorBlock=extra_sc/Delay_discrete/OFF Delay  TreatAsAtomicUnit=on
  Unit Delay : UnitDelay  X0=ic  SampleTime=Ts
  either edge : Constant  Value=[1 1]
  neg. edge : Constant  Value=[0 1]
  pos. edge : Constant  Value=[1 0]
  Out : Outport
  wires:
  either edge/1 -> Multiport Switch/4
  Demux/2 -> NEGATIVE Edge/Enable
  Demux/1 -> POSITIVE Edge/Enable
  Multiport Switch/1 -> Demux/1
  Constant1/1 -> Multiport Switch/1
  neg. edge/1 -> Multiport Switch/3
  pos. edge/1 -> Multiport Switch/2
  In/1 -> Unit Delay/1, NEGATIVE Edge/1(IN), POSITIVE Edge/1(IN)
  Unit Delay/1 -> NEGATIVE Edge/2(IN previous), POSITIVE Edge/2(IN previous)
  POSITIVE Edge/1(OUT) -> Logical Operator1/1
  NEGATIVE Edge/1(OUT) -> Logical Operator1/2
  Logical Operator1/1 -> Out/1

== system powerlib_extras/Discrete  Control Blocks/Discrete On/Off Delay/OFF Delay ==
  IN : Inport  Port=1  LatchInput=off
  DELAY : Inport  Port=2  LatchInput=off
  Enable : EnablePort
  Constant2 : Constant  Value=-Ts
  Constant3 : Constant  Value=Ts
  Discrete Edge Detector : powerlib_extras/Discrete  Control Blocks/Discrete Edge Detector  model=Falling  ic=ic  Ts=Ts
  Logical Operator1 : Logic
  Logical Operator2 : Logic  Operator=NOT
  Logical Operator3 : Logic  Operator=NOT
  Relational Operator : RelationalOperator  LogicOutDataTypeMode=Boolean  InputSameDT=on
  Sum1 : Sum  Inputs=+-  SaturateOnIntegerOverflow=on  InputSameDT=on
  Switch : Switch  Threshold=0.5  SaturateOnIntegerOverflow=on  InputSameDT=on
  Unit Delay : UnitDelay  Orientation=left  SampleTime=Ts
  OUT : Outport
  wires:
  Unit Delay/1 -> Switch/3
  Sum1/1 -> Relational Operator/2, Unit Delay/1
  Switch/1 -> Sum1/1
  Constant3/1 -> Sum1/2
  Relational Operator/1 -> Logical Operator1/2
  IN/1 -> Discrete Edge Detector/1, Logical Operator2/1
  Logical Operator1/1 -> Logical Operator3/1
  DELAY/1 -> Switch/1
  Discrete Edge Detector/1 -> Switch/2
  Constant2/1 -> Relational Operator/1
  Logical Operator2/1 -> Logical Operator1/1
  Logical Operator3/1 -> OUT/1

== system powerlib_extras/Discrete  Control Blocks/Discrete On/Off Delay/ON Delay ==
  IN : Inport  Port=1  LatchInput=off
  DELAY : Inport  Port=2  LatchInput=off
  Enable : EnablePort
  Constant2 : Constant  Value=-Ts
  Constant3 : Constant  Value=Ts
  Discrete Edge Detector : powerlib_extras/Discrete  Control Blocks/Discrete Edge Detector  model=Rising  ic=ic  Ts=Ts
  Logical Operator1 : Logic
  Relational Operator : RelationalOperator  LogicOutDataTypeMode=Boolean  InputSameDT=on
  Sum1 : Sum  Inputs=+-  SaturateOnIntegerOverflow=on  InputSameDT=on
  Switch : Switch  Threshold=0.5  SaturateOnIntegerOverflow=on  InputSameDT=on
  Unit Delay : UnitDelay  Orientation=left  SampleTime=Ts
  OUT : Outport
  wires:
  Unit Delay/1 -> Switch/3
  Sum1/1 -> Unit Delay/1, Relational Operator/2
  Switch/1 -> Sum1/1
  Constant3/1 -> Sum1/2
  Relational Operator/1 -> Logical Operator1/2
  IN/1 -> Discrete Edge Detector/1, Logical Operator1/1
  Logical Operator1/1 -> OUT/1
  DELAY/1 -> Switch/1
  Discrete Edge Detector/1 -> Switch/2
  Constant2/1 -> Relational Operator/1
